simulink model "DC_Motor_Speed"  (R2020b)
settings: Solver=VariableStepAuto  StartTime=0.0  StopTime=10.0  RelTol=1e-3
undefined symbols (not defined in the file): b, J, K, L, R
settings Model: Creator=intel  LastModifiedBy=intel

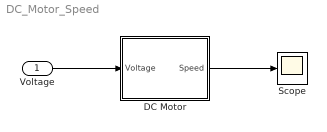
== system DC_Motor_Speed ==
  Voltage : Inport
  DC Motor : Subsystem
  Scope : Scope
  wires:
  Voltage/1 -> DC Motor/1(Voltage)
  DC Motor/1(Speed) -> Scope/1

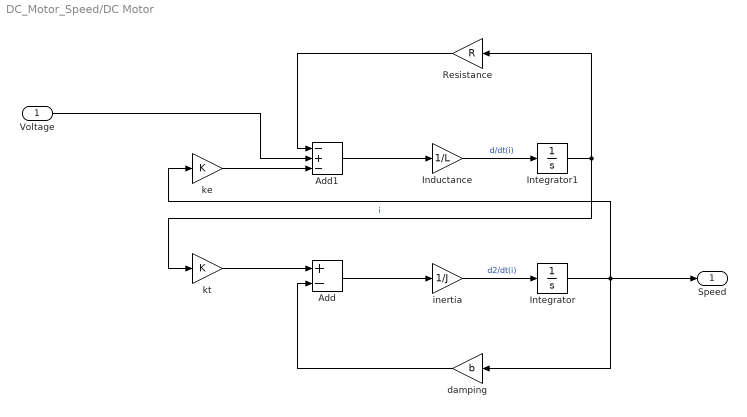
== system DC_Motor_Speed/DC Motor ==
  Voltage : Inport
  Add : Sum  Inputs=+-
  Add1 : Sum  Inputs=-+-
  Inductance : Gain  Gain=1/L
  Integrator : Integrator
  Integrator1 : Integrator
  Resistance : Gain  Gain=R
  damping : Gain  Gain=b
  inertia : Gain  Gain=1/J
  ke : Gain  Gain=K
  kt : Gain  Gain=K
  Speed : Outport
  wires:
  Integrator/1 -> Speed/1, ke/1, damping/1
  ke/1 -> Add1/3
  Voltage/1 -> Add1/2
  Inductance/1 -> Integrator1/1  "d/dt(i)"
  Integrator1/1 -> Resistance/1, kt/1  "i"
  damping/1 -> Add/2
  Add/1 -> inertia/1
  Resistance/1 -> Add1/1
  Add1/1 -> Inductance/1
  inertia/1 -> Integrator/1  "d2/dt(i)"
  kt/1 -> Add/1
